simulink model "test_maxon_driver"  (R2020a)
settings: Solver=FixedStepAuto  StartTime=0.0  StopTime=inf  FixedStep=1  RelTol=1e-3
libraries: lib2020a_maxon x1
settings Model: EnablePacing=on  Creator=ugurm  LastModifiedBy=ugurm

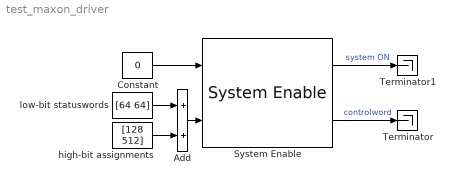
== system test_maxon_driver ==
  Add : Sum
  Constant : Constant  Value=0
  System Enable : lib2020a_maxon/System Enable  SystemSampleTime=-1  Latency=0  AutoFrameSizeCalculation=off
  Terminator : Terminator
  Terminator1 : Terminator
  high-bit assignments : Constant  Value=[128 512]
  low-bit statuswords : Constant  Value=[64 64]
  wires:
  Constant/1 -> System Enable/1
  low-bit statuswords/1 -> Add/1
  System Enable/2 -> Terminator/1  "controlword"
  System Enable/1 -> Terminator1/1  "system ON"
  Add/1 -> System Enable/2
  high-bit assignments/1 -> Add/2
